simulink model "triad_activation_dynamic_test"  (R2018b)
settings: Solver=FixedStepAuto  StartTime=0.0  StopTime=100  FixedStep=fswParams.sample_time_s  RelTol=1e-3
libraries: TriadActivation_lib x1
settings Model: Creator=Taylor  LastModifiedBy=Taylor

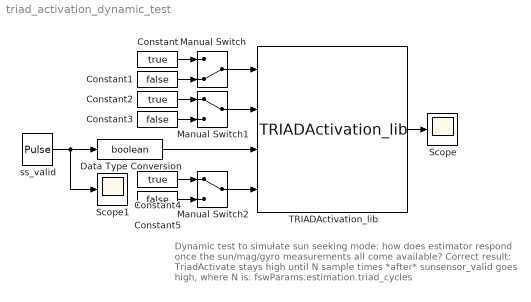
== system triad_activation_dynamic_test ==
  note: Dynamic test to simulate sun seeking mode: how does estimator
      | respond once the sun/mag/gyro measurements all come available?
      |
      | Correct result: TriadActivate stays high until N sample times *after*
      | sunsensor_valid goes high, where N is:
      |
      | fswParams.estimation.triad_cycles
  Constant : Constant  Value=true
  Constant1 : Constant  Value=false
  Constant2 : Constant  Value=true
  Constant3 : Constant  Value=false
  Constant4 : Constant  Value=true
  Constant5 : Constant  Value=false
  Data Type Conversion : DataTypeConversion  OutDataTypeStr=boolean
  Manual Switch : ManualSwitch  CurrentSetting=0
  Manual Switch1 : ManualSwitch
  Manual Switch2 : ManualSwitch
  Scope : Scope
  Scope1 : Scope
  TRIADActivation_lib : TriadActivation_lib/TRIADActivation_lib  SystemSampleTime=-1
  ss_valid : DiscretePulseGenerator  PulseType=Time based  Period=50  PulseWidth=25  PhaseDelay=5
  wires:
  Constant/1 -> Manual Switch/1
  Constant1/1 -> Manual Switch/2
  Constant2/1 -> Manual Switch1/1
  Constant3/1 -> Manual Switch1/2
  Manual Switch/1 -> TRIADActivation_lib/1
  Manual Switch1/1 -> TRIADActivation_lib/2
  ss_valid/1 -> Scope1/1, Data Type Conversion/1
  Constant5/1 -> Manual Switch2/2
  Constant4/1 -> Manual Switch2/1
  Manual Switch2/1 -> TRIADActivation_lib/4
  Data Type Conversion/1 -> TRIADActivation_lib/3
  TRIADActivation_lib/1 -> Scope/1
